simulink library "LibCrossAr_v2020a"  (R2020a)
settings: Solver=FixedStepDiscrete  StartTime=0.0  StopTime=inf  RelTol=1e-3
undefined symbols (not defined in the file or in its folder): ModelParam
Description:
  | % Francesco Conti, Gaetano Scarano, Stefania Colonnese, Mauro Biagi, 2021/01/04%
  | % Copyright: This is published under BSD BSD 3-Clause License
  | 
  | % Copyright (c) 2021, francescoconti748 (Francesco Conti)
  | % All rights reserved, see LICENSE file
  | %
settings Model: Creator=gscarano  LastModifiedBy=conti
settings DataIOCC: LimitDataPoints=on  SaveFormat=Array  SignalLoggingSaveFormat=ModelDataLogs  SaveOutput=off  SignalLogging=off  SaveTime=off  ReturnWorkspaceOutputs=off
settings OptimizationCC: ExpressionDepthLimit=2147483647  LifeSpan=inf
settings DebuggingCC: AlgebraicLoopMsg=error  UnderspecifiedInitializationDetection=Classic  MergeDetectMultiDrivingBlocksExec=none  SolverPrmCheckMsg=warning  SingleTaskRateTransMsg=error  FcnCallInpInsideContextMsg=warning  StateNameClashWarn=warning  SFUnexpectedBacktrackingDiag=warning  SFNoUnconditionalDefaultTransitionDiag=warning  SFExecutionAtInitializationDiag=none  ArithmeticOperatorsInVariantConditions=warning
settings HardwareCC: ProdBitPerPointer=32  ProdBitPerSizeT=32  ProdBitPerPtrDiffT=32  ProdLargestAtomicFloat=None  ProdIntDivRoundTo=Undefined  ProdEndianess=Unspecified  ProdWordSize=32  ProdHWDeviceType=32-bit Generic
settings ModelReferenceCC: PropagateSignalLabelsOutOfModel=off
settings SFSimCC: SimUseLocalCustomCode=off  CustomCodeUndefinedFunction=UseInterfaceOnly
settings RTWCC: RTWUseLocalCustomCode=off
settings CodeAppCC: StateflowObjectComments=on
settings GRTTargetCC: TargetLangStandard=C89/C90 (ANSI)  CombineOutputUpdateFcns=off  GRTInterface=on
settings ConfigComp: CovMetricSettings=dw  CovSaveCumulativeToWorkspaceVar=on  CovSaveSingleToWorkspaceVar=on  CovExternalEMLEnable=off

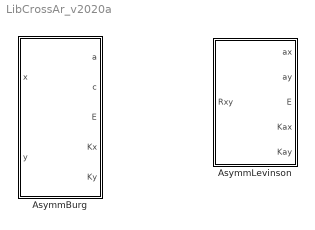
== system LibCrossAr_v2020a ==
  AsymmBurg : Subsystem  Description=|  mask{N=ModelParam.Nlags, Samples4Frame=ModelParam.Samples4Frame}
      | % Francesco Conti, Gaetano Scarano, Stefania Colonnese, Mauro Biagi, 2021/01/04%
      | % Copyright: This is published under BSD BSD 3-Clause License
      | 
      | % Copyright (c) 2021, francescoconti748 (Francesco Conti)
      | % All rights reserved, see LICENSE file
      | %
  AsymmLevinson : Subsystem  Description=|  mask{Nlags=ModelParam.Nlags, Samples4Frame=0}
      | % Francesco Conti, Gaetano Scarano, Stefania Colonnese, Mauro Biagi, 2021/01/04%
      | % Copyright: This is published under BSD BSD 3-Clause License
      | 
      | % Copyright (c) 2021, francescoconti748 (Francesco Conti)
      | % All rights reserved, see LICENSE file
      | %

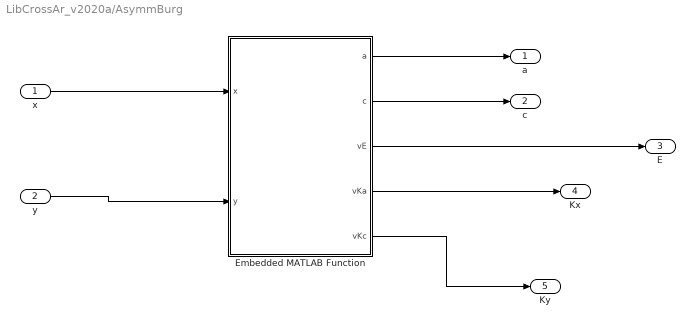
== system LibCrossAr_v2020a/AsymmBurg ==
  x : Inport
  y : Inport  Port=2
  Embedded MATLAB Function : MATLAB Function  Description=|  TreatAsAtomicUnit=on
      | % Francesco Conti, Gaetano Scarano, Stefania Colonnese, Mauro Biagi, 2021/01/04%
      | % Copyright: This is published under BSD BSD 3-Clause License
      | 
      | % Copyright (c) 2021, francescoconti748 (Francesco Conti)
      | % All rights reserved, see LICENSE file
      | %
  a : Outport
  c : Outport  Port=2
  E : Outport  Port=3
  Kx : Outport  Port=4
  Ky : Outport  Port=5
  wires:
  Embedded MATLAB Function/4(vKa) -> Kx/1
  Embedded MATLAB Function/3(vE) -> E/1
  Embedded MATLAB Function/5(vKc) -> Ky/1
  y/1 -> Embedded MATLAB Function/2(y)
  x/1 -> Embedded MATLAB Function/1(x)
  Embedded MATLAB Function/2(c) -> c/1
  Embedded MATLAB Function/1(a) -> a/1

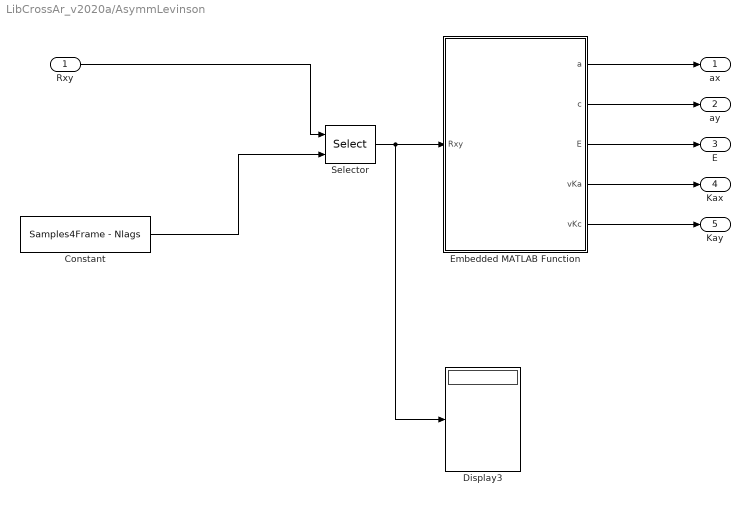
== system LibCrossAr_v2020a/AsymmLevinson ==
  Rxy : Inport
  Constant : Constant  Value=Samples4Frame - Nlags
  Display3 : Display
  Embedded MATLAB Function : MATLAB Function  TreatAsAtomicUnit=on
  Selector : Selector  IndexOptions=Starting index (port)  Indices=[1 3]  OutputSizes=2*Nlags+1
  ax : Outport
  ay : Outport  Port=2
  E : Outport  Port=3
  Kax : Outport  Port=4
  Kay : Outport  Port=5
  wires:
  Rxy/1 -> Selector/1
  Constant/1 -> Selector/2
  Selector/1 -> Display3/1, Embedded MATLAB Function/1(Rxy)
  Embedded MATLAB Function/1(a) -> ax/1
  Embedded MATLAB Function/2(c) -> ay/1
  Embedded MATLAB Function/3(E) -> E/1
  Embedded MATLAB Function/4(vKa) -> Kax/1
  Embedded MATLAB Function/5(vKc) -> Kay/1

== matlab function LibCrossAr_v2020a/AsymmBurg/Embedded MATLAB Function ==
  data: a output; c output; vE output; x input; vKa output; vKc output; y input; N parameter int32
function [a, c, vE, vKa, vKc] = gBurg_Kxycoeff(x,y,N)

% Francesco Conti, Gaetano Scarano, Stefania Colonnese, Mauro Biagi, 2021/01/04%
% Copyright: This is published under BSD BSD 3-Clause License

% Copyright (c) 2021, francescoconti748 (Francesco Conti)
% All rights reserved, see LICENSE file
%


 L = numel(x);

 vKc  = double(zeros(N,1)); %Ka vector
 vKa  = double(zeros(N,1)); %Kc vector
 vE   = double(zeros(N+1,1)); %knwon terms vector, feeding sequence power estimates
 
 % 0-th iteration
 fx = x;
 fy = y;
 
 bx = x;
 by = y;
 
  a  = zeros(N+1,1);
 c = zeros(N+1,1);
  a(1)  = 1;
 c(N+1) = 1;
 
 
 vE(1) = (x'*y) / L; %initialization
 %
 for j=1:N
     j1 = j + 1;
     jf = j1;
     jb = j;
     num_c = fx(jf:end)'  * by(jb:end-1); 
     num_a = fy(jf:end)'  * bx(jb:end-1);
     %
     Den = (fx(jf:end)'*fy(jf:end) + bx(jb:end-1)'*by(jb:end-1) ) ;
     %
     Kc = -2.* num_c ./ Den;
     Ka = -2.* num_a ./ Den;
     %
     vKc(j) = Kc;
     vKa(j) = Ka;
     %
     fxprev = fx;
     fyprev = fy;
     
     %residual errors update
     fx(jf:end)= fxprev(jf:end) + Kc*bx(jb:end-1);
     fy(jf:end)= fyprev(jf:end) + Ka*by(jb:end-1);
     bx(jf:end)= Ka*fxprev(jf:end) + bx(jb:end-1);
     by(jf:end)= Kc*fyprev(jf:end) + by(jb:end-1);
     
     %
     vE(j1) = vE(j) * (1-Kc*Ka);
     %
     %vE(j1) = abs(sqrt(real((fx(j1+1:end)'*fy(j1+1:end)) * (bx(j1:end-1)'*by(j1:end-1))))) /(L);
     
     
     asaved  = a;
          
     a(1:j+1)= asaved(1:j+1) + Kc * c(N+1-j:end);
     c(N+1-j:end) = Ka* asaved(1:j+1) +      c(N+1-j:end);
     
 end
end

== matlab function LibCrossAr_v2020a/AsymmLevinson/Embedded MATLAB Function ==
  data: Rxy input; a output; c output; E output; vKa output; vKc output
function [a, c, E, vKa, vKc] = glAsymmLevinson(Rxy)
% Francesco Conti, Gaetano Scarano, Stefania Colonnese, Mauro Biagi, 2021/01/04%
% Copyright: This is published under BSD BSD 3-Clause License

% Copyright (c) 2021, francescoconti748 (Francesco Conti)
% All rights reserved, see LICENSE file
%
 % check numel(Rxy) is odd
 
 N = int32((numel(Rxy)-1)/2);
 vKa   = zeros(N,1); %vector containing Ka
 vKc  = zeros(N,1); %vector containing Kc
 
 a  = zeros(N+1,1); %estimated coeffs a
 c = zeros(N+1,1); %estimated coeffs a
 %
 rxy   = Rxy(N+2:end); %cross-corr, positive lags
 ryx  =  Rxy(N:-1:1); %cross-corr, negative lags
 %
 %coeff initialization
 a(1)  = 1;
 c(N+1) = 1;
 
 % first iteration
 E = Rxy(N+1); %cross-power, initialization
 %
 % iterative system solution, AR order n
 for n=1:N
     %
     Kc = -  (rxy(n:-1:1)'  * a(1:n))/E; 
     Ka = - (ryx(1:n)'   * c(N+1-(n-1):end))/E;
     %
     vKa(n)  = Ka;
     vKc(n) = Kc;
     %
     E = E * (1-Kc*Ka); %known term update
     %
     asaved  = a;
     %
     a(1:n+1)      =      asaved(1:n+1) + Kc * c(N+1-n:end); %coeffs a update
     c(N+1-n:end) = Ka* asaved(1:n+1) +      c(N+1-n:end); %coeff c update
 end
end
%
